simulink subsystem "WDN_safety_controller"  (R2022b)
settings: Solver=VariableStepAuto  StartTime=0.0  StopTime=inf  RelTol=1e-3
model mask{consumer_tank_max=550, consumer_tank_min=100, pump_tank_min=150}
  mask prompts: consumer_tank_max "consumer tank_max [mm]"; consumer_tank_min "consumer tank min [mm]"; pump_tank_min "pump_tank_min [mm]"
libraries: simulink x6
settings Model: DefaultTestHarness=Return_water_and_safety_controller_Harness2  Creator=laula  LastModifiedBy=laula

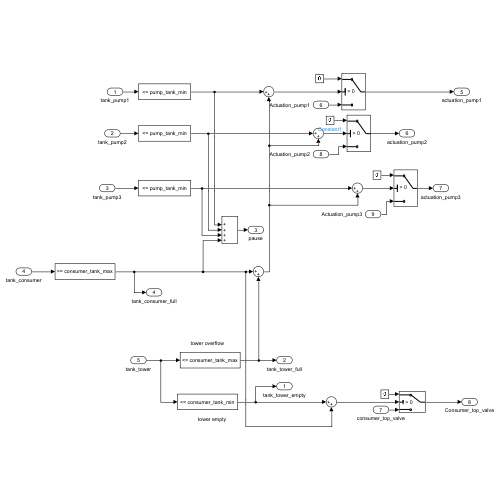
[thumbnail: Simulink's stored preview of the top-level diagram]
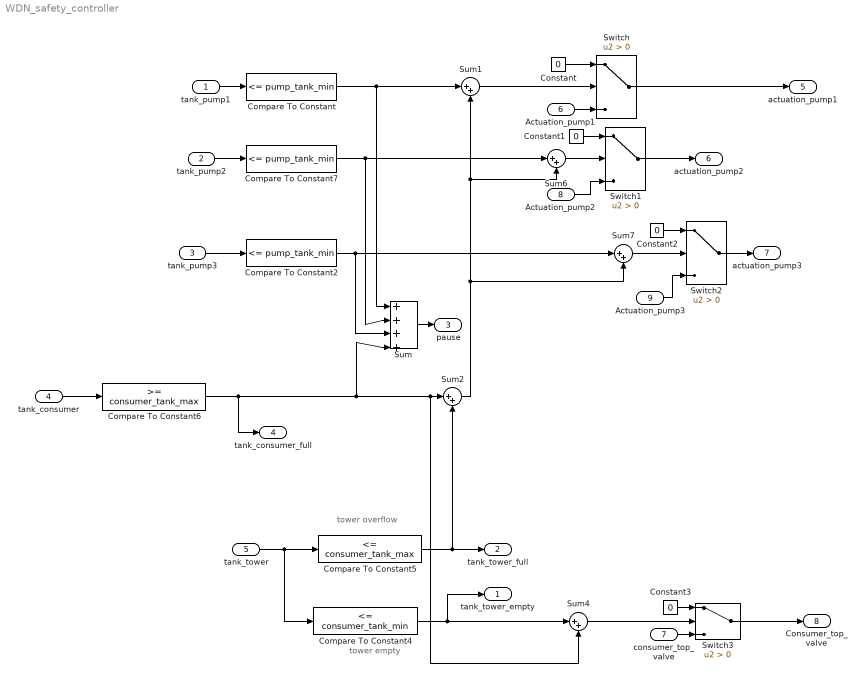
== system WDN_safety_controller ==
  note: tower overflow
  note: tower empty
  tank_pump1 : Inport
  tank_pump2 : Inport  Port=2
  tank_pump3 : Inport  Port=3
  tank_consumer : Inport  Port=4
  tank_tower : Inport  Port=5
  Actuation_pump1 : Inport  Port=6
  consumer_top_valve : Inport  Port=7
  Actuation_pump2 : Inport  Port=8
  Actuation_pump3 : Inport  Port=9
  Compare To Constant : simulink/Logic and Bit Operations/Compare To Constant  relop=<=  const=pump_tank_min  OutDataTypeStr=boolean
  Compare To Constant2 : simulink/Logic and Bit Operations/Compare To Constant  relop=<=  const=pump_tank_min  OutDataTypeStr=boolean
  Compare To Constant4 : simulink/Logic and Bit Operations/Compare To Constant  relop=<=  const=consumer_tank_min  OutDataTypeStr=boolean
  Compare To Constant5 : simulink/Logic and Bit Operations/Compare To Constant  relop=<=  const=consumer_tank_max  OutDataTypeStr=boolean
  Compare To Constant6 : simulink/Logic and Bit Operations/Compare To Constant  relop=>=  const=consumer_tank_max  OutDataTypeStr=boolean
  Compare To Constant7 : simulink/Logic and Bit Operations/Compare To Constant  relop=<=  const=pump_tank_min  OutDataTypeStr=boolean
  Constant{,1..3} (4 alike) : Constant  Value=0
  Sum : Sum  Inputs=|++++
  Sum{1..2,4,6..7} (5 alike) : Sum  Inputs=|++
  Switch{,1..3} (4 alike) : Switch  Criteria=u2 > Threshold  SaturateOnIntegerOverflow=off  InputSameDT=off
  tank_tower_empty : Outport
  tank_tower_full : Outport  Port=2
  pause : Outport  Description=|  Port=3
      | If pause is high, return water system can not keep up. Pause controllers, wait for singal to go low
      | 
      | Alternatively, tower tank is close to overflow
  tank_consumer_full : Outport  Port=4
  actuation_pump1 : Outport  Port=5
  actuation_pump2 : Outport  Port=6
  actuation_pump3 : Outport  Port=7
  Consumer_top_valve : Outport  Port=8
  wires:
  tank_pump1/1 -> Compare To Constant/1
  tank_pump3/1 -> Compare To Constant2/1
  Switch/1 -> actuation_pump1/1
  tank_tower/1 -> Compare To Constant4/1, Compare To Constant5/1
  Compare To Constant4/1 -> Sum4/1, tank_tower_empty/1
  Switch3/1 -> Consumer_top_valve/1
  tank_consumer/1 -> Compare To Constant6/1
  Sum4/1 -> Switch3/2
  Compare To Constant6/1 -> Sum4/2, Sum2/1, Sum/4, tank_consumer_full/1
  Compare To Constant/1 -> Sum/1, Sum1/1
  Sum1/1 -> Switch/2
  Compare To Constant5/1 -> Sum2/2, tank_tower_full/1
  Switch1/1 -> actuation_pump2/1
  Constant1/1 -> Switch1/1
  Sum6/1 -> Switch1/2
  tank_pump2/1 -> Compare To Constant7/1
  Compare To Constant7/1 -> Sum/2, Sum6/1
  Switch2/1 -> actuation_pump3/1
  Constant2/1 -> Switch2/1
  Actuation_pump2/1 -> Switch1/3
  Actuation_pump3/1 -> Switch2/3
  Sum7/1 -> Switch2/2
  Compare To Constant2/1 -> Sum/3, Sum7/1
  Sum2/1 -> Sum7/2, Sum6/2, Sum1/2
  Sum/1 -> pause/1
  Actuation_pump1/1 -> Switch/3
  Constant/1 -> Switch/1
  consumer_top_valve/1 -> Switch3/3
  Constant3/1 -> Switch3/1
